simulink model "SampleSimulinkModel"  (Simulink 7.0)
settings: Solver=ode45  StartTime=0.0  StopTime=10.0  RelTol=1e-3
undefined symbols (not defined in the file or in its folder): ts
libraries: dspmlti4 x1
settings Model: Creator=Bais  LastModifiedBy=Bais

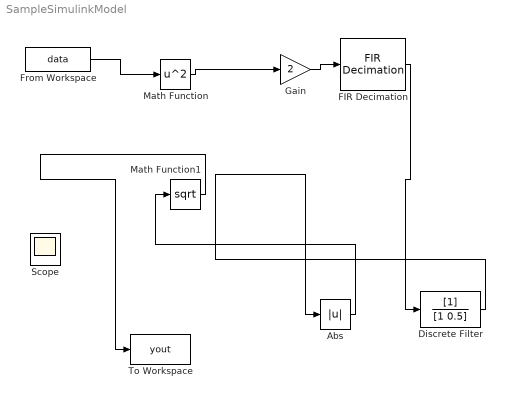
== system SampleSimulinkModel ==
  Abs : Abs  OutDataType=sfix(16)  OutScaling=2^0
  Discrete Filter : DiscreteFilter  Denominator=[1 0.5]
  FIR Decimation : dspmlti4/FIR Decimation  DialogController=dspdialog.FIRDecimation  DialogControllerArgs=DataTag0  h=fir1(35,0.4)  D=15  filtStruct=Direct form  framing=Maintain input frame size  outputBufInitCond=0  roundingMode=Floor  overflowMode=off  FilterSource=Specify via dialog  FilterObject=Hm_firdecim
  From Workspace : FromWorkspace  VariableName=data  SampleTime=ts
  Gain : Gain  Gain=2  ParameterDataType=sfix(16)  ParameterScaling=2^0  OutDataType=sfix(16)  OutScaling=2^0
  Math Function : Math  Operator=square  OutDataType=sfix(16)  OutScaling=2^0  SaturateOnIntegerOverflow=on
  Math Function1 : Math  Operator=sqrt  OutDataType=sfix(16)  OutScaling=2^0  SaturateOnIntegerOverflow=on
  Scope : Scope
  To Workspace : ToWorkspace  VariableName=yout  SampleTime=-1  SaveFormat=Structure
  wires:
  From Workspace/1 -> Math Function/1
  Math Function/1 -> Gain/1
  Gain/1 -> FIR Decimation/1
  FIR Decimation/1 -> Discrete Filter/1
  Discrete Filter/1 -> Abs/1
  Abs/1 -> Math Function1/1
  Math Function1/1 -> To Workspace/1
